simulink model "normal_linear"  (R2016b)
settings: Solver=VariableStepAuto  StartTime=0.0  StopTime=10.0  RelTol=1e-3
undefined symbols (not defined in the file): A, B, C
settings Model: Creator=Amin  LastModifiedBy=Amin

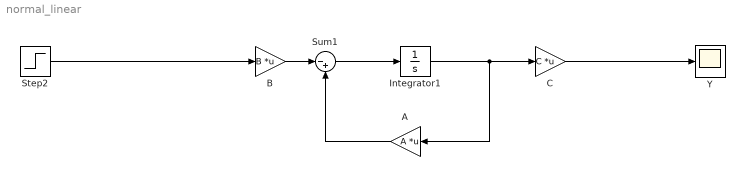
== system normal_linear ==
  A : Gain  Gain=A  Multiplication=Matrix(K*u)
  B : Gain  Gain=B  Multiplication=Matrix(K*u)
  C : Gain  Gain=C  Multiplication=Matrix(K*u)
  Integrator1 : Integrator  InitialCondition=[0.3 0 0 0]
  Step2 : Step  After=3  SampleTime=0
  Sum1 : Sum  Inputs=|-+
  Y : Scope
  wires:
  C/1 -> Y/1
  Integrator1/1 -> C/1, A/1
  A/1 -> Sum1/2
  Sum1/1 -> Integrator1/1
  B/1 -> Sum1/1
  Step2/1 -> B/1
